simulink model "FPR_Demo"  (R2023a)
settings: Solver=FixedStepAuto  StartTime=0.0  StopTime=604800  FixedStep=10  RelTol=1e-3
settings Model: Creator=Owner  LastModifiedBy=Owner

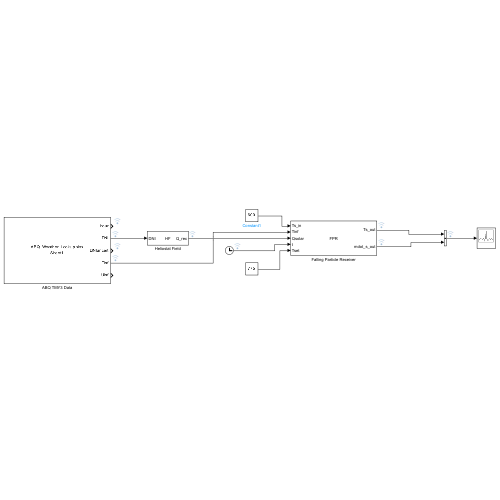
[thumbnail: Simulink's stored preview of the top-level diagram]
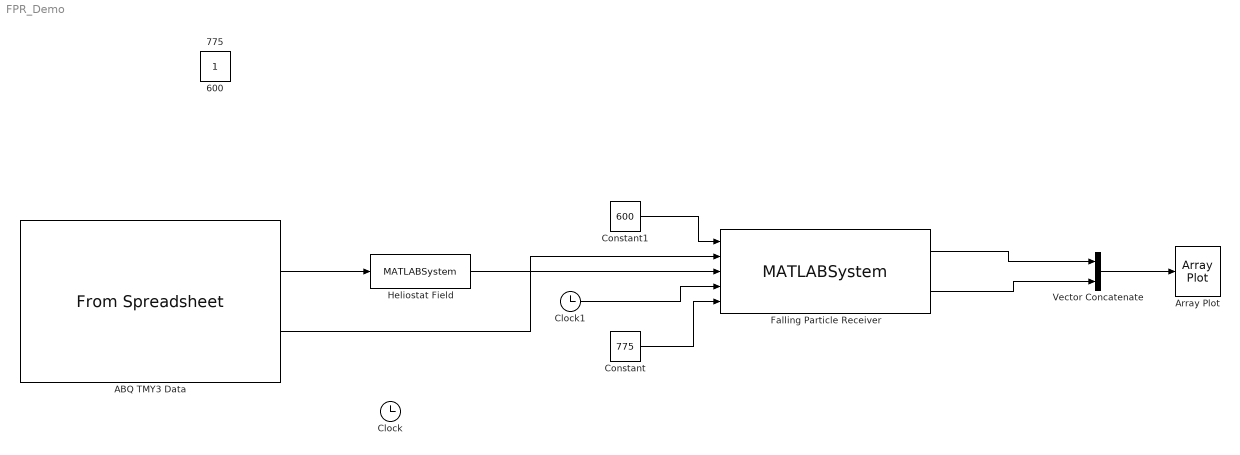
== system FPR_Demo ==
  ABQ TMY3 Data : FromSpreadsheet  FileName=ABQ_Weather_Lookup.xlsx  OutDataTypeStr=double
  Array Plot : ArrayPlot  WindowPosition=[1014.000000,178.000000,800.000000,500.000000,]  ScopeFrameLocation=window  YLimits=[-2.0692,18.6228]
  Clock1 : Clock
  Constant : Constant  Value=775
  Constant1 : Constant  Value=600
  Falling Particle Receiver : MATLABSystem  System=FPR  H=1.2  W=1.2  d=0.0417  SimulateUsing=Code generation  Ts0=600  hInf=5  cp_s=1250  rho_s=3500  phi_s=0.6  epsilon_s=0.88  alpha_s=0.92  tauLag=1500  tauLead=100
      mask Type: FPR
      mask Display:
      | disp('FPR');
      | port_label('input',1,'Ts_in');
      | port_label('input',2,'Tinf');
      | port_label('input',3,'Qsolar');
      | port_label('input',4,'t');
      | port_label('input',5,'Tset');
      | port_label('output',1,'Ts_out');
      | port_label('output',2,'mdot_s_out');
  Heliostat Field : MATLABSystem  System=HF  n=150  H=5  W=5  eta_op=0.6  SimulateUsing=Code generation
      mask Type: HF
      mask Display:
      | disp('HF');
      | port_label('input',1,'DNI');
      | port_label('output',1,'Q_rec');
  Vector Concatenate : Concatenate
  600 : Constant  IOType=siggen
  775 : Constant  IOType=siggen
  Clock : Clock
      settings: IOType=siggen
  wires:
  Heliostat Field/1 -> Falling Particle Receiver/3
  Constant/1 -> Falling Particle Receiver/5
  Clock1/1 -> Falling Particle Receiver/4
  Constant1/1 -> Falling Particle Receiver/1
  Falling Particle Receiver/1 -> Vector Concatenate/1
  Falling Particle Receiver/2 -> Vector Concatenate/2
  Vector Concatenate/1 -> Array Plot/1
  ABQ TMY3 Data/2 -> Heliostat Field/1
  ABQ TMY3 Data/4 -> Falling Particle Receiver/2
